simulink model "QFproof"  (R2020b)
settings: Solver=FixedStepAuto  StartTime=0.0  StopTime=15  FixedStep=0.02  RelTol=1e-3
libraries: powerlib x1
settings Model: Creator=许丹阳  LastModifiedBy=许丹阳

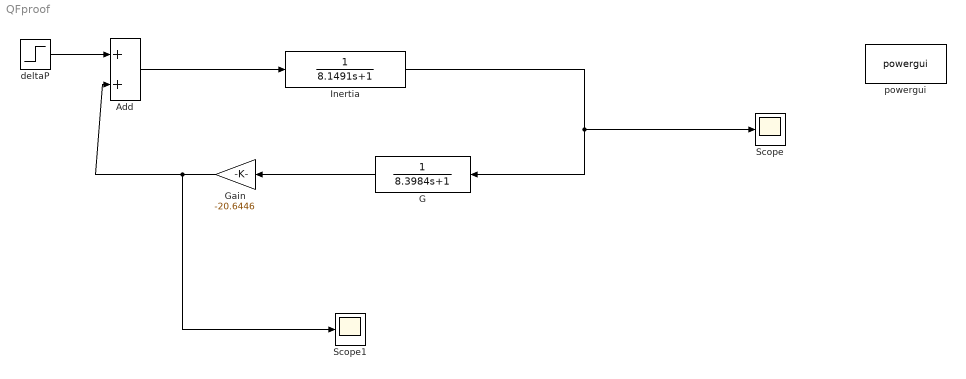
== system QFproof ==
  Add : Sum
  G : TransferFcn  Numerator=[0,1]  Denominator=[8.3984,1]
  Gain : Gain  Gain=-20.6446
  Inertia : TransferFcn  Denominator=[8.1491,1]
  Scope : Scope
  Scope1 : Scope
  deltaP : Step  Time=0  After=-0.11213  SampleTime=0
  powergui : powerlib/powergui  Priority=1  SimulationMode=Continuous  SampleTime=1e-12  frequency=60  Iterations=50  frequencyindice=60  Pbase=100e6  ErrMax=1e-4  UnitsV=kV  UnitsW=MW  buscounter=0  FunctionMessages=off  echomessages=off  EnableUseOfTLC=off  CurrentSourceSwitches=off  DisableSnubberDevices=off  DisableRonSwitches=off  DisableVfSwitches=off  DisplayEquations=off  AutomaticDiscreteSolvers=off  SolverType=Tustin/Backward Euler (TBE)  Interpol=off  ExternalGateDelay=off  methode=off  Ts=100  x0status=blocks  SPID=on  SwTol=0  HookPort=off  NonlinearTolerance=1e-4  nMaxIteration=100  ContinueOnMaxIteration=off  RestoreLinks=warning  ResistiveCurrentMeasurement=off  Frange=[0:2:500]  Ylog=off  Xlog=on  ShowGrid=off  save=off  variable=ZData  structure=0  ZoomFFT=off  StartTime=0.0  cycles=1  DisplayStyle=1  fundamental=60  FreqAxis=off  MaxFrequency=1000  frequencyindicesteady=1  RmsSteady=1  display=off
  wires:
  G/1 -> Gain/1
  Add/1 -> Inertia/1
  Inertia/1 -> Scope/1, G/1
  deltaP/1 -> Add/1
  Gain/1 -> Scope1/1, Add/2
